simulink model "single_phase_hafewave_controle_Rectifier"  (R2020a)
settings: Solver=VariableStepAuto  StartTime=0.0  StopTime=.05  RelTol=1e-3
libraries: powerlib x24
settings Model: Creator=hp  LastModifiedBy=hp

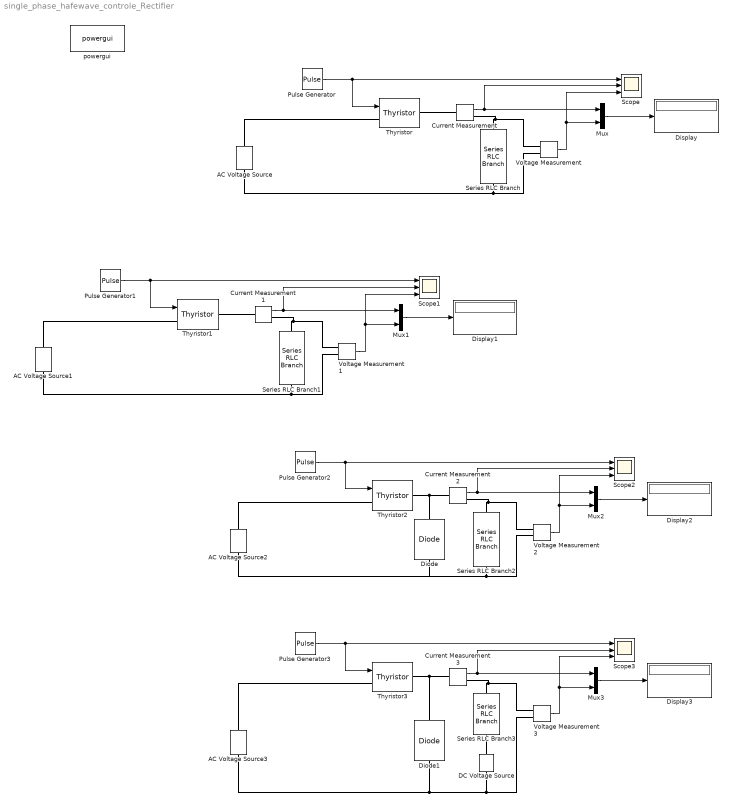
== system single_phase_hafewave_controle_Rectifier ==
  AC Voltage Source{,1..3} (4 alike) : powerlib/Electrical Sources/AC Voltage Source  Amplitude=100  Phase=0  Frequency=50  SampleTime=0  Measurements=None  BusType=swing  Pref=10e3  Qref=0  Qmin=-inf  Qmax=+inf
  Current Measurement{,1..3} (4 alike) : powerlib/Measurements/Current Measurement  PhasorSimulation=off  OutputType=Complex  PSBequivalent=0
  DC Voltage Source : powerlib/Electrical Sources/DC Voltage Source  Amplitude=40  Measurements=None
  Diode : powerlib/Power Electronics/Diode  Ron=0.001  Lon=0  Vf=0.8  IC=0  UseSnubber=0  Rs=500  Cs=250e-9  Measurements=off
  Diode1 : powerlib/Power Electronics/Diode  Ron=0.001  Lon=0  Vf=0.8  IC=0  UseSnubber=0  Rs=500  Cs=250e-9  Measurements=off
  Display{,1..3} (4 alike) : Display
  Mux{,1..3} (4 alike) : Mux  Inputs=2
  Pulse Generator : DiscretePulseGenerator  PulseType=Time based  Period=1/50  PulseWidth=5  PhaseDelay=30/(360*50)
  Pulse Generator1 : DiscretePulseGenerator  PulseType=Time based  Period=1/50  PulseWidth=5  PhaseDelay=30/(360*50)
  Pulse Generator2 : DiscretePulseGenerator  PulseType=Time based  Period=1/50  PulseWidth=5  PhaseDelay=30/(360*50)
  Pulse Generator3 : DiscretePulseGenerator  PulseType=Time based  Period=1/50  PulseWidth=5  PhaseDelay=90/(360*50)
  Scope{,1..3} (4 alike) : Scope  NumInputPorts=3
  Series RLC Branch : powerlib/Elements/Series RLC Branch  LConnTagsString=__new0  RConnTagsString=__new0  BranchType=R  Resistance=10  Inductance=1e-3  SetiL0=off  InitialCurrent=0  Capacitance=1e-6  Setx0=off  InitialVoltage=0  Measurements=None
  Series RLC Branch1 : powerlib/Elements/Series RLC Branch  LConnTagsString=__new0  RConnTagsString=__new0  BranchType=RL  Resistance=10  Inductance=5e-3  SetiL0=off  InitialCurrent=0  Capacitance=1e-6  Setx0=off  InitialVoltage=0  Measurements=None
  Series RLC Branch2 : powerlib/Elements/Series RLC Branch  LConnTagsString=__new0  RConnTagsString=__new0  BranchType=RL  Resistance=10  Inductance=5e-3  SetiL0=off  InitialCurrent=0  Capacitance=1e-6  Setx0=off  InitialVoltage=0  Measurements=None
  Series RLC Branch3 : powerlib/Elements/Series RLC Branch  LConnTagsString=__new0  RConnTagsString=__new0  BranchType=RL  Resistance=10  Inductance=1e-3  SetiL0=off  InitialCurrent=0  Capacitance=1e-6  Setx0=off  InitialVoltage=0  Measurements=None
  Thyristor{,1..3} (4 alike) : powerlib/Power Electronics/Thyristor  Ron=0.001  Lon=0  Vf=0.8  IC=0  Rs=500  Cs=250e-9  Measurements=off
  Voltage Measurement{,1..3} (4 alike) : powerlib/Measurements/Voltage Measurement  PhasorSimulation=off  OutputType=Complex  PSBequivalent=0
  powergui : powerlib/powergui  Priority=1  SimulationMode=Discrete  SampleTime=50e-6  frequency=60  Iterations=50  frequencyindice=0  Pbase=100e6  ErrMax=1e-4  UnitsV=kV  UnitsW=MW  buscounter=0  FunctionMessages=off  echomessages=off  EnableUseOfTLC=off  CurrentSourceSwitches=off  DisableSnubberDevices=off  DisableRonSwitches=off  DisableVfSwitches=off  DisplayEquations=off  AutomaticDiscreteSolvers=off  SolverType=Tustin/Backward Euler (TBE)  Interpol=off  ExternalGateDelay=off  methode=off  Ts=100  x0status=blocks  SPID=on  SwTol=0  HookPort=off  NonlinearTolerance=1e-4  nMaxIteration=100  ContinueOnMaxIteration=off  RestoreLinks=warning  ResistiveCurrentMeasurement=off  Frange=[0:2:500]  Ylog=off  Xlog=on  ShowGrid=off  save=off  variable=ZData  structure=0  ZoomFFT=off  StartTime=0.0  cycles=1  DisplayStyle=1  fundamental=60  FreqAxis=off  MaxFrequency=1000  frequencyindicesteady=1  RmsSteady=1  display=off
  wires:
  Pulse Generator/1 -> Scope/1, Thyristor/1
  Current Measurement/1 -> Mux/1, Scope/2
  Voltage Measurement/1 -> Mux/2, Scope/3
  Mux/1 -> Display/1
  Pulse Generator1/1 -> Scope1/1, Thyristor1/1
  Voltage Measurement1/1 -> Mux1/2, Scope1/3
  Mux1/1 -> Display1/1
  Current Measurement1/1 -> Mux1/1, Scope1/2
  Current Measurement2/1 -> Mux2/1, Scope2/2
  Mux2/1 -> Display2/1
  Pulse Generator2/1 -> Scope2/1, Thyristor2/1
  Voltage Measurement2/1 -> Mux2/2, Scope2/3
  Current Measurement3/1 -> Mux3/1, Scope3/2
  Mux3/1 -> Display3/1
  Pulse Generator3/1 -> Scope3/1, Thyristor3/1
  Voltage Measurement3/1 -> Mux3/2, Scope3/3
  connections:
  AC Voltage Source/RConn1 -- Thyristor/LConn1
  Series RLC Branch/LConn1 -- Current Measurement/RConn1 -- Voltage Measurement/LConn1
  Series RLC Branch/RConn1 -- AC Voltage Source/LConn1 -- Voltage Measurement/LConn2
  Current Measurement/LConn1 -- Thyristor/RConn1
  Series RLC Branch1/RConn1 -- AC Voltage Source1/LConn1 -- Voltage Measurement1/LConn2
  Series RLC Branch1/LConn1 -- Current Measurement1/RConn1 -- Voltage Measurement1/LConn1
  AC Voltage Source1/RConn1 -- Thyristor1/LConn1
  Current Measurement1/LConn1 -- Thyristor1/RConn1
  Series RLC Branch2/RConn1 -- Diode/LConn1 -- AC Voltage Source2/LConn1 -- Voltage Measurement2/LConn2
  Series RLC Branch2/LConn1 -- Current Measurement2/RConn1 -- Voltage Measurement2/LConn1
  AC Voltage Source2/RConn1 -- Thyristor2/LConn1
  Current Measurement2/LConn1 -- Diode/RConn1 -- Thyristor2/RConn1
  Voltage Measurement3/LConn2 -- DC Voltage Source/LConn1 -- Diode1/LConn1 -- AC Voltage Source3/LConn1
  Series RLC Branch3/LConn1 -- Current Measurement3/RConn1 -- Voltage Measurement3/LConn1
  AC Voltage Source3/RConn1 -- Thyristor3/LConn1
  Current Measurement3/LConn1 -- Diode1/RConn1 -- Thyristor3/RConn1
  DC Voltage Source/RConn1 -- Series RLC Branch3/RConn1
